simulink model "draft7"  (R2023a)
settings: Solver=VariableStepAuto  StartTime=0.0  StopTime=10  FixedStep=0.0001  MaxStep=0.1  RelTol=1e-3  AbsTol=1e-3  EnableMultiTasking=on
model workspace (MAT data in the model file):
  C_Gimbal = 0.1
  C_IAP = 0.01
  IAP_Pa = 0
  K_Gimbal = 0
  K_IAP = 10
  LeftAbdominalMuscleForce = 0
  LeftBackMuscleForce = 0
  LeftTransverse1MuscleForce = 0
  LeftTransverse2MuscleForce = 0
  Moment_AR = 0
  Moment_FE = 0
  Moment_LB = 0
  RightAbdominalMuscleForce = 0
  RightBackMuscleForce = 0
  RightTransverse1MuscleForce = 0
  RightTransverse2MuscleForce = 0
  a = 1
  b = 1
undefined symbols (not defined in the file): X, Y, Z
libraries: sm_lib x279, nesl_utility x233, simulink_extras x33, checkpacklib x3, simulink x1
(part 1 of 7)
settings Model: PacingRate=0.110000  Creator=Siril TD  LastModifiedBy=siril
settings SolverCC: AutoScaleAbsTol=off  ZeroCrossAlgorithm=Adaptive  AlgebraicLoopSolver=TrustRegion
settings DataIOCC: LimitDataPoints=on  MaxDataPoints=10000  ReturnWorkspaceOutputsName=SDOSimTest_Log
settings OptimizationCC: LifeSpan=inf
settings DebuggingCC: ReadBeforeWriteMsg=DisableAll  WriteAfterWriteMsg=DisableAll  WriteAfterReadMsg=DisableAll  IgnoredZcDiagnostic=none  MultiTaskDSMMsg=none  UnconnectedInputMsg=warning  UnconnectedOutputMsg=warning  UnconnectedLineMsg=warning  AllowSymbolicDim=off  SFUnexpectedBacktrackingDiag=warning  SFNoUnconditionalDefaultTransitionDiag=warning  SFExecutionAtInitializationDiag=none  ArithmeticOperatorsInVariantConditions=warning
settings ModelReferenceCC: EnableRefExpFcnMdlSchedulingChecks=on
settings SFSimCC: SimUseLocalCustomCode=off  CustomCodeUndefinedFunction=UseInterfaceOnly
settings RTWCC: RTWUseLocalCustomCode=off  DLArmComputeVersion=19.05
settings CodeAppCC: StateflowObjectComments=on
settings GRTTargetCC: TargetLangStandard=C89/C90 (ANSI)
settings ConfigComp: CovMetricSettings=dw  CovSaveCumulativeToWorkspaceVar=on  CovSaveSingleToWorkspaceVar=on  CovExternalEMLEnable=off  CovSFcnEnable=off
settings SimscapeCC: SimscapeLogType=all  SimscapeLogSimulationStatistics=on  SimscapeLogDataHistory=10000

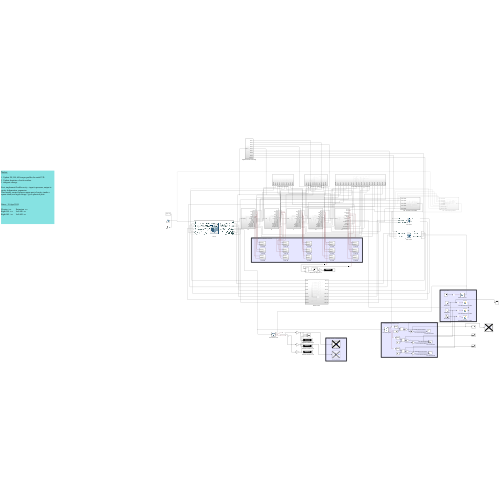
[thumbnail: Simulink's stored preview of the top-level diagram]
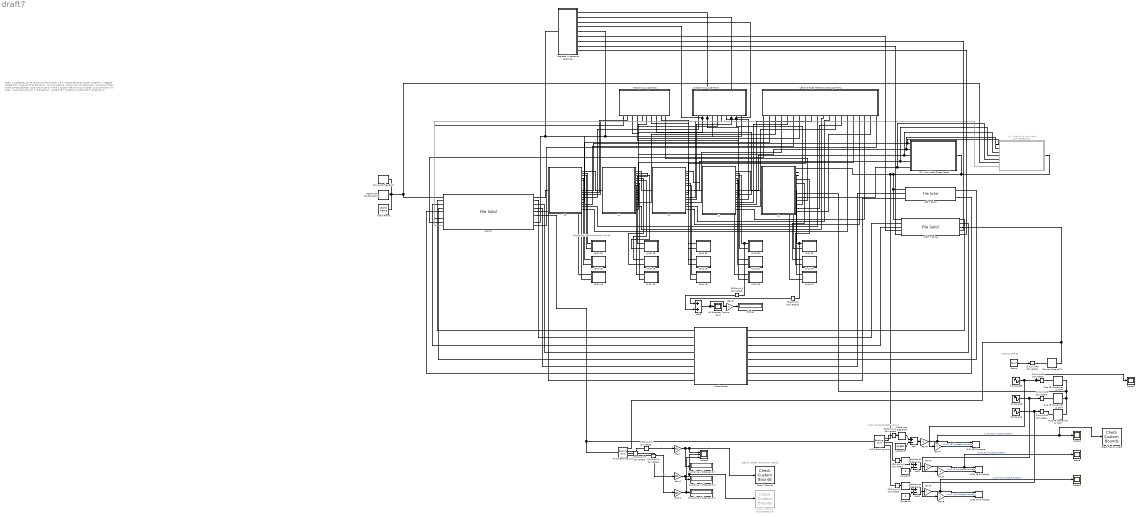
== system draft7 ==
  note: Segmental Moment-Rotation Curves
  note: L1-S1 Moment-Rotation Curve
  note: Loading Profiles
  note: Stability Check - Plumbline method
  note: Notes:
      |
      | 1. Update FE, LB, AR torque profiles for each IVD
      | 2. Update densities of each vertebra
      | 3. integrate ribcage
      |
      | First, implement flexible cavity - input is pressure, output is cavity deformation, expansion
      | Then model contact between upper part of cavity (make a square shaft) and rigid ribcage - give spherical joint
      |
      | Notes : 19-Apr-2024
      |
      | Flexion +ve Extension -ve
      | Right LB +ve Left LB -ve
      | Right AR +ve Left AR -ve
  Add : Sum  Inputs=+-
  Add1 : Sum  Inputs=+-
  Add2 : Sum  Inputs=+-
  Add3 : Sum
  Check Flexion Angle : checkpacklib/Check Custom Bounds  InstantiateOnLoad=on  enabled=off  stopWhenAssertionFail=off  export=off  ViewDlgPos=[100 200 510 390]  OpenViewOnLoad=off  LaunchViewOnOpen=off  TimeUnits=seconds  EnableUpperBound=on  UpperBoundTimes=[5 10]  UpperBoundAmplitudes=[51 51];  EnableLowerBound=on  LowerBoundTimes=[6 10]  LowerBoundAmplitudes=[49 49];
      settings: LibrarySourceBlock=sdolib/Signal Constraints/Check Custom Bounds
  Check X Bounds : checkpacklib/Check Custom Bounds  InstantiateOnLoad=on  enabled=off  stopWhenAssertionFail=off  export=off  ViewDlgPos=[622 345 510 390]  OpenViewOnLoad=off  LaunchViewOnOpen=off  TimeUnits=seconds  EnableUpperBound=on  UpperBoundTimes=[0 10]  UpperBoundAmplitudes=[2 2];  EnableLowerBound=on  LowerBoundTimes=[0 10]  LowerBoundAmplitudes=[-2 -2]
      settings: LibrarySourceBlock=sdolib/Signal Constraints/Check Custom Bounds
  Check Y Bounds : checkpacklib/Check Custom Bounds  Commented=on  InstantiateOnLoad=on  enabled=off  stopWhenAssertionFail=off  export=off  ViewDlgPos=[509 222 510 390]  OpenViewOnLoad=off  LaunchViewOnOpen=off  TimeUnits=seconds  EnableUpperBound=on  UpperBoundTimes=[0 10]  UpperBoundAmplitudes=[2 2];  EnableLowerBound=on  LowerBoundTimes=[0 10]  LowerBoundAmplitudes=[-2 -2]
      settings: LibrarySourceBlock=sdolib/Signal Constraints/Check Custom Bounds
  Constant2 : Constant  Value=14.555
  Constant3 : Constant  Value=0
  Constant4 : Constant  Value=0
  Display : Display
      settings: Decimation=2
  Flexion force at T1 : sm_lib/Forces and Torques/External Force and Torque  ForceResolutionFrame=AttachedFrame  EnableForceX=off  EnableForceY=on  EnableForceZ=off  EnableForce=off  TorqueResolutionFrame=AttachedFrame  EnableTorqueX=off  EnableTorqueY=off  EnableTorqueZ=off  EnableTorque=off
  Gain : Gain  Gain=100
  Gain1 : Gain  Gain=100
  Gain2 : Gain  Gain=100
  Gain{3..4,6..7} (4 alike) : Gain  Gain=-1
  Gain5 : Gain
  Gain8 : Gain
  Gain9 : Gain
  IAP - Individual Forces Model : Subsystem
  IAP - Internal Springs Model : Subsystem  Commented=on
  IAP Extensor Torque at L3 : Scope
  Interspinous Ligaments : Subsystem
  L1 : Subsystem
  L1-L2 AR : Subsystem
  L1-L2 FE : Subsystem
  L1-L2 LB : Subsystem
  L1-S1 AR Simscape : Record  FileSettingsInternal="{\"entries\":[{\"content\":{\"excelSettings\":{\"content\":{},\"type\":\"Streamout.ExcelSettings\"}},\"type\":\"Streamout.FileSettingStorage\",\"uuid\":\"c761fec1-51ad-4fdc-aadc-7a7c0ed1755e\"}],\"packageUris\":[\"http://schema.mathworks.com/mf0/streamout_blocks/R2020a\"],\"version\":\"1.0\"}"  Layout=[1 1]  SignalsInternal="{\"entries\":[{\"content\":{\"signals\":[{\"content\":{\"blockPath\":[\"draft7/L1-S1 AR Simscape\"],\"dimensions\":[1,1],\"domain\":\"draft7/L1-S1 AR Simscape\",\"lineColor\":\"#d95319\",\"port\":1,\"sid\":[\"\"],\"signalID\":183,\"signalName\":\"L1-S1 AR Simscape Rotation\"},\"type\":\"RecordBlkView.Signal\",\"uuid\":\"264051fc-ffd2-4aa6-9d28-74edf75983d9\"},{\"content\":{\"blockPath\":[\"draft7/L1-S1 AR Simscape\"],\"dimensions\":[1],\"domain\":\"draft7/L1-S1 AR Simscape\",\"lineColor\":\"#edb120\",\"port\":2,\"sid\":[\"\"],\"signalID\":187,\"signalName\":\"L1-S1 AR Simscape Moment\"},\"type\":\"RecordBlkView.Signal\",\"uuid\":\"a252a67f-d163-4ee1-9bea-fb1124a7b68d\"}]},\"type\":\"RecordBlkView.InputSignals\",\"uuid\":\"d04fa92a-6ab9-41c9-bd02-3e9af83bab1f\"}],\"packageUris\":[\"http://schema.mathworks.com/mf0/streamout_blocks/R2020a\"],\"version\":\"1.0\"}"  VisualizationBindings="{\"xyplotplugin\":{\"info\":[{\"series\":[],\"subplotID\":1}]}}"  CompatibilityTag=XY
  L1-S1 Bushing Joint : sm_lib/Joints/Bushing Joint  JointMode=Normal  SenseConstraintForce=off  SenseConstraintForceX=off  SenseConstraintForceY=off  SenseConstraintForceZ=off  SenseConstraintTorque=off  SenseConstraintTorqueX=off  SenseConstraintTorqueY=off  SenseConstraintTorqueZ=off  SenseTotalForce=off  SenseTotalForceX=off  SenseTotalForceY=off  SenseTotalForceZ=off  SenseTotalTorque=off  SenseTotalTorqueX=off  SenseTotalTorqueY=off  SenseTotalTorqueZ=off  CompositeWrenchDir=FollowerOnBase  CompositeWrenchFrame=FollowerFrame  PxEquilibriumPosition=0  PxEquilibriumPositionUnits=m  PxSpringStiffness=0  PxSpringStiffnessUnits=N/m  PxDampingCoefficient=0  PxDampingCoefficientUnits=N/(m/s)  PxTorqueActuationMode=NoTorque  PxMotionActuationMode=ComputedMotion  PxSensePosition=off  PxSenseVelocity=off  PxSenseAcceleration=off  PxSenseTorqueForce=off  PxSenseLowerLimitTorqueForce=off  PxSenseUpperLimitTorqueForce=off  PxLowerLimitSpecify=off  PxLowerLimitBound=-1  PxLowerLimitBoundUnits=m  PxLowerLimitStiffness=1e6  PxLowerLimitStiffnessUnits=N/m  PxLowerLimitDamping=1e3  PxLowerLimitDampingUnits=N/(m/s)  PxLowerLimitTransitionRegionWidth=1e-4  PxLowerLimitTransitionRegionWidthUnits=m  PxUpperLimitSpecify=off  PxUpperLimitBound=1  PxUpperLimitBoundUnits=m  PxUpperLimitStiffness=1e6  PxUpperLimitStiffnessUnits=N/m  PxUpperLimitDamping=1e3  PxUpperLimitDampingUnits=N/(m/s)  PxUpperLimitTransitionRegionWidth=1e-4  PxUpperLimitTransitionRegionWidthUnits=m  PxPositionTargetSpecify=off  PxPositionTargetPriority=High  PxPositionTargetValue=0  PxPositionTargetValueUnits=m  PxVelocityTargetSpecify=off  PxVelocityTargetPriority=High  PxVelocityTargetValue=0  PxVelocityTargetValueUnits=m/s  PyEquilibriumPosition=0  PyEquilibriumPositionUnits=m  PySpringStiffness=0  PySpringStiffnessUnits=N/m  PyDampingCoefficient=0  PyDampingCoefficientUnits=N/(m/s)  PyTorqueActuationMode=NoTorque  PyMotionActuationMode=ComputedMotion  PySensePosition=off  PySenseVelocity=off  PySenseAcceleration=off  PySenseTorqueForce=off  PySenseLowerLimitTorqueForce=off  PySenseUpperLimitTorqueForce=off  PyLowerLimitSpecify=off  PyLowerLimitBound=-1  PyLowerLimitBoundUnits=m  PyLowerLimitStiffness=1e6  PyLowerLimitStiffnessUnits=N/m  PyLowerLimitDamping=1e3  PyLowerLimitDampingUnits=N/(m/s)  PyLowerLimitTransitionRegionWidth=1e-4  PyLowerLimitTransitionRegionWidthUnits=m  PyUpperLimitSpecify=off  PyUpperLimitBound=1  PyUpperLimitBoundUnits=m  PyUpperLimitStiffness=1e6  PyUpperLimitStiffnessUnits=N/m  PyUpperLimitDamping=1e3  PyUpperLimitDampingUnits=N/(m/s)  PyUpperLimitTransitionRegionWidth=1e-4  PyUpperLimitTransitionRegionWidthUnits=m  PyPositionTargetSpecify=off  PyPositionTargetPriority=High  PyPositionTargetValue=0  PyPositionTargetValueUnits=m  PyVelocityTargetSpecify=off  PyVelocityTargetPriority=High  PyVelocityTargetValue=0  PyVelocityTargetValueUnits=m/s  PzEquilibriumPosition=0  PzEquilibriumPositionUnits=m  PzSpringStiffness=0  PzSpringStiffnessUnits=N/m  PzDampingCoefficient=0  PzDampingCoefficientUnits=N/(m/s)  PzTorqueActuationMode=NoTorque  PzMotionActuationMode=ComputedMotion  PzSensePosition=off  PzSenseVelocity=off  PzSenseAcceleration=off  PzSenseTorqueForce=off  PzSenseLowerLimitTorqueForce=off  PzSenseUpperLimitTorqueForce=off  PzLowerLimitSpecify=off  PzLowerLimitBound=-1  PzLowerLimitBoundUnits=m  PzLowerLimitStiffness=1e6  PzLowerLimitStiffnessUnits=N/m  PzLowerLimitDamping=1e3  PzLowerLimitDampingUnits=N/(m/s)  PzLowerLimitTransitionRegionWidth=1e-4  PzLowerLimitTransitionRegionWidthUnits=m  PzUpperLimitSpecify=off  PzUpperLimitBound=1  PzUpperLimitBoundUnits=m  PzUpperLimitStiffness=1e6  PzUpperLimitStiffnessUnits=N/m  PzUpperLimitDamping=1e3  PzUpperLimitDampingUnits=N/(m/s)  PzUpperLimitTransitionRegionWidth=1e-4  PzUpperLimitTransitionRegionWidthUnits=m  PzPositionTargetSpecify=off  PzPositionTargetPriority=High  PzPositionTargetValue=0  PzPositionTargetValueUnits=m  PzVelocityTargetSpecify=off  PzVelocityTargetPriority=High  PzVelocityTargetValue=0  PzVelocityTargetValueUnits=m/s  RxEquilibriumPosition=0  RxEquilibriumPositionUnits=deg  RxSpringStiffness=0  RxSpringStiffnessUnits=N*m/deg  RxDampingCoefficient=0  RxDampingCoefficientUnits=N*m/(deg/s)  RxTorqueActuationMode=NoTorque  RxMotionActuationMode=ComputedMotion  RxSensePosition=on  RxSenseVelocity=off  RxSenseAcceleration=off  RxSenseTorqueForce=off  RxSenseLowerLimitTorqueForce=off  RxSenseUpperLimitTorqueForce=off  RxLowerLimitSpecify=off  RxLowerLimitBound=-90  RxLowerLimitBoundUnits=deg  RxLowerLimitStiffness=1e4  RxLowerLimitStiffnessUnits=N*m/deg  RxLowerLimitDamping=10  RxLowerLimitDampingUnits=N*m/(deg/s)  RxLowerLimitTransitionRegionWidth=0.1  RxLowerLimitTransitionRegionWidthUnits=deg  RxUpperLimitSpecify=off  RxUpperLimitBound=90  RxUpperLimitBoundUnits=deg  RxUpperLimitStiffness=1e4  RxUpperLimitStiffnessUnits=N*m/deg  RxUpperLimitDamping=10  RxUpperLimitDampingUnits=N*m/(deg/s)  RxUpperLimitTransitionRegionWidth=0.1  RxUpperLimitTransitionRegionWidthUnits=deg  RxPositionTargetSpecify=off  RxPositionTargetPriority=High  RxPositionTargetValue=0  RxPositionTargetValueUnits=deg  RxVelocityTargetSpecify=off  RxVelocityTargetPriority=High  RxVelocityTargetValue=0  RxVelocityTargetValueUnits=deg/s  RyEquilibriumPosition=0  RyEquilibriumPositionUnits=deg  RySpringStiffness=0  RySpringStiffnessUnits=N*m/deg  RyDampingCoefficient=0  RyDampingCoefficientUnits=N*m/(deg/s)  RyTorqueActuationMode=NoTorque  RyMotionActuationMode=ComputedMotion  RySensePosition=on  RySenseVelocity=off  RySenseAcceleration=off  RySenseTorqueForce=off  RySenseLowerLimitTorqueForce=off  RySenseUpperLimitTorqueForce=off  RyLowerLimitSpecify=off  RyLowerLimitBound=-90  RyLowerLimitBoundUnits=deg  RyLowerLimitStiffness=1e4  RyLowerLimitStiffnessUnits=N*m/deg  RyLowerLimitDamping=10  RyLowerLimitDampingUnits=N*m/(deg/s)  RyLowerLimitTransitionRegionWidth=0.1  RyLowerLimitTransitionRegionWidthUnits=deg  RyUpperLimitSpecify=off  RyUpperLimitBound=90  RyUpperLimitBoundUnits=deg  RyUpperLimitStiffness=1e4  RyUpperLimitStiffnessUnits=N*m/deg  RyUpperLimitDamping=10  RyUpperLimitDampingUnits=N*m/(deg/s)  RyUpperLimitTransitionRegionWidth=0.1  RyUpperLimitTransitionRegionWidthUnits=deg  RyPositionTargetSpecify=off  RyPositionTargetPriority=High  RyPositionTargetValue=0  RyPositionTargetValueUnits=deg  RyVelocityTargetSpecify=off  RyVelocityTargetPriority=High  RyVelocityTargetValue=0  RyVelocityTargetValueUnits=deg/s  RzEquilibriumPosition=0  RzEquilibriumPositionUnits=deg  RzSpringStiffness=0  RzSpringStiffnessUnits=N*m/deg  RzDampingCoefficient=0  RzDampingCoefficientUnits=N*m/(deg/s)  RzTorqueActuationMode=NoTorque  RzMotionActuationMode=ComputedMotion  RzSensePosition=on  RzSenseVelocity=off  RzSenseAcceleration=off  RzSenseTorqueForce=off  RzSenseLowerLimitTorqueForce=off  RzSenseUpperLimitTorqueForce=off  RzLowerLimitSpecify=off  RzLowerLimitBound=-90  RzLowerLimitBoundUnits=deg  RzLowerLimitStiffness=1e4  RzLowerLimitStiffnessUnits=N*m/deg  RzLowerLimitDamping=10  RzLowerLimitDampingUnits=N*m/(deg/s)  RzLowerLimitTransitionRegionWidth=0.1  RzLowerLimitTransitionRegionWidthUnits=deg  RzUpperLimitSpecify=off  RzUpperLimitBound=90  RzUpperLimitBoundUnits=deg  RzUpperLimitStiffness=1e4  RzUpperLimitStiffnessUnits=N*m/deg  RzUpperLimitDamping=10  RzUpperLimitDampingUnits=N*m/(deg/s)  RzUpperLimitTransitionRegionWidth=0.1  RzUpperLimitTransitionRegionWidthUnits=deg  RzPositionTargetSpecify=off  RzPositionTargetPriority=High  RzPositionTargetValue=0  RzPositionTargetValueUnits=deg  RzVelocityTargetSpecify=off  RzVelocityTargetPriority=High  RzVelocityTargetValue=0  RzVelocityTargetValueUnits=deg/s
  L1-S1 FE Simscape : Record  FileSettingsInternal="{\"entries\":[{\"content\":{\"excelSettings\":{\"content\":{},\"type\":\"Streamout.ExcelSettings\"}},\"type\":\"Streamout.FileSettingStorage\",\"uuid\":\"9db1673e-bbaa-437a-8537-4e772d2a90f6\"}],\"packageUris\":[\"http://schema.mathworks.com/mf0/streamout_blocks/R2020a\"],\"version\":\"1.0\"}"  Layout=[1 1]  SignalsInternal="{\"entries\":[{\"content\":{\"signals\":[{\"content\":{\"blockPath\":[\"draft7/L1-S1 FE Simscape\"],\"dimensions\":[1,1],\"domain\":\"draft7/L1-S1 FE Simscape\",\"lineColor\":\"#ff13a6\",\"port\":1,\"sid\":[\"\"],\"signalID\":167,\"signalName\":\"L1-S1 FE Simscape Rotation\"},\"type\":\"RecordBlkView.Signal\",\"uuid\":\"c1594988-5f2b-4ea3-9ef2-5b94fe21d5f8\"},{\"content\":{\"blockPath\":[\"draft7/L1-S1 FE Simscape\"],\"dimensions\":[1],\"domain\":\"draft7/L1-S1 FE Simscape\",\"lineColor\":\"#fe330a\",\"port\":2,\"sid\":[\"\"],\"signalID\":171,\"signalName\":\"L1-S1 FE Simscape Moment\"},\"type\":\"RecordBlkView.Signal\",\"uuid\":\"b92ce8fd-0f35-4184-b4f5-937e9b6e7470\"}]},\"type\":\"RecordBlkView.InputSignals\",\"uuid\":\"db540f72-e83b-464a-95e3-44d444f527ba\"}],\"packageUris\":[\"http://schema.mathworks.com/mf0/streamout_blocks/R2020a\"],\"version\":\"1.0\"}"  VisualizationBindings="{\"xyplotplugin\":{\"info\":[{\"series\":[],\"subplotID\":1}]}}"  CompatibilityTag=XY
  L1-S1 LB Simscape : Record  FileSettingsInternal="{\"entries\":[{\"content\":{\"excelSettings\":{\"content\":{},\"type\":\"Streamout.ExcelSettings\"}},\"type\":\"Streamout.FileSettingStorage\",\"uuid\":\"68995d24-6116-4abf-89ba-75caefee83bb\"}],\"packageUris\":[\"http://schema.mathworks.com/mf0/streamout_blocks/R2020a\"],\"version\":\"1.0\"}"  Layout=[1 1]  SignalsInternal="{\"entries\":[{\"content\":{\"signals\":[{\"content\":{\"blockPath\":[\"draft7/L1-S1 LB Simscape\"],\"dimensions\":[1,1],\"domain\":\"draft7/L1-S1 LB Simscape\",\"lineColor\":\"#22b573\",\"port\":1,\"sid\":[\"\"],\"signalID\":175,\"signalName\":\"L1-S1 LB Simscape Rotation\"},\"type\":\"RecordBlkView.Signal\",\"uuid\":\"30783bb8-1c86-4cdf-87e2-2a28f747091a\"},{\"content\":{\"blockPath\":[\"draft7/L1-S1 LB Simscape\"],\"dimensions\":[1],\"domain\":\"draft7/L1-S1 LB Simscape\",\"lineColor\":\"#0072bd\",\"port\":2,\"sid\":[\"\"],\"signalID\":179,\"signalName\":\"L1-S1 LB Simscape Moment\"},\"type\":\"RecordBlkView.Signal\",\"uuid\":\"2a8f21ee-91f9-4dc2-9379-b6999c3c9a9c\"}]},\"type\":\"RecordBlkView.InputSignals\",\"uuid\":\"a080d18d-00c5-434d-a6df-27a9e497c067\"}],\"packageUris\":[\"http://schema.mathworks.com/mf0/streamout_blocks/R2020a\"],\"version\":\"1.0\"}"  VisualizationBindings="{\"xyplotplugin\":{\"info\":[{\"series\":[],\"subplotID\":1}]}}"  CompatibilityTag=XY
  L2 : Subsystem
  L2-L3 AR : Subsystem
  L2-L3 FE : Subsystem
  L2-L3 LB : Subsystem
  L3 : Subsystem
  L3-L4 AR : Subsystem
  L3-L4 FE : Subsystem
  L3-L4 LB : Subsystem
  L4 : Subsystem
  L4-L5  AR : Subsystem
  L4-L5  FE : Subsystem
  L4-L5  LB : Subsystem
  L5 : Subsystem
  L5-S1 AR : Subsystem
  L5-S1 FE : Subsystem
  L5-S1 LB : Subsystem
  Left T Spine : sm_lib/Body Elements/File Solid  ExtGeomFileName=C:\Users\siril\OneDrive\Desktop\TIM-Control\Matlab\Simscape models\CAD - with COM\SymmetricModel\draft7\LeftThoracicSpineWithRibcage.step  UnitType=FromFile  ExtGeomFileUnits=m  StepReaderType=HEX  ExportConvexHullGeometry=off  InertiaType=CalculateFromGeometry  Mass=1  MassUnits=kg  CenterOfMass=[0 0 0]  CenterOfMassUnits=m  MomentsOfInertia=[1 1 1]  MomentsOfInertiaUnits=kg*m^2  ProductsOfInertia=[0 0 0]  ProductsOfInertiaUnits=kg*m^2  BasedOnType=Density  Density=0.182  DensityUnits=g/cm^3  DoExposeReferenceFrame=off  SerializedFrames=<Frames><Frame><Id>Frame1</Id><Value><Name>To L1</Name><Origin><Source>GeometricFeature</Source><FeatureName>segment 762</FeatureName></Origin><PrimaryAxis><DefinedDirection>-Z</DefinedDirection><Source>GeometricFeature</Source><SourceDirection>+Z</SourceDirection><FeatureName>planar surface 1266</FeatureName></PrimaryAxis><SecondaryAxis><DefinedDirection>+X</DefinedDirection><Source>ReferenceFrame</Source><SourceDirection>+X</SourceDirection><FeatureName></FeatureName></SecondaryAxis></Value></Frame><Frame><Id>Frame2</Id><Value><Name>To Left Abdominal Muscle</Name><Origin><Source>GeometricFeature</Source><FeatureName>planar surface 54556</FeatureName></Origin><PrimaryAxis><DefinedDirection>+Z</DefinedDirection><Source>GeometricFeature</Source><SourceDirection>+Z</SourceDirection><FeatureName>planar surface 54556</FeatureName></PrimaryAxis><SecondaryAxis><DefinedDirection>+X</DefinedDirection><Source>ReferenceFrame</Source><SourceDirection>+X</SourceDirection><FeatureName></FeatureName></SecondaryAxis></Value></Frame><Frame><Id>Frame3</Id><Value><Name>To Left Back Muscle</Name><Origin><Source>GeometricFeature</Source><FeatureName>planar surface 54574</FeatureName></Origin><PrimaryAxis><DefinedDirection>-Z</DefinedDirection><Source>GeometricFeature</Source><SourceDirection>+Z</SourceDirection><FeatureName>planar surface 54574</FeatureName></PrimaryAxis><SecondaryAxis><DefinedDirection>+X</DefinedDirection><Source>ReferenceFrame</Source><SourceDirection>+X</SourceDirection><FeatureName></FeatureName></SecondaryAxis></Value></Frame><Frame><Id>Frame4</Id><Value><Name>To Left Transverse1 Muscle</Name><Origin><Source>GeometricFeature</Source><FeatureName>planar surface 54586</FeatureName></Origin><PrimaryAxis><DefinedDirection>+Z</DefinedDirection><Source>GeometricFeature</Source><SourceDirection>+Z</SourceDirection><FeatureName>planar surface 54586</FeatureName></PrimaryAxis><SecondaryAxis><DefinedDirection>+X</DefinedDirection><Source>ReferenceFrame</Source><SourceDirection>+X</SourceDirection><FeatureName></FeatureName></SecondaryAxis></Value></Frame><Frame><Id>Frame5</Id><Value><Name>To Left Transverse2 Muscle</Name><Origin><Source>GeometricFeature</Source><FeatureName>planar surface 54611</FeatureName></Origin><PrimaryAxis><DefinedDirection>+Z</DefinedDirection><Source>GeometricFeature</Source><SourceDirection>+Z</SourceDirection><FeatureName>planar surface 54611</FeatureName></PrimaryAxis><SecondaryAxis><DefinedDirection>+X</DefinedDirection><Source>ReferenceFrame</Source><SourceDirection>+X</SourceDirection><FeatureName></FeatureName></SecondaryAxis></Value></Frame></Frames>  GraphicType=FromGeometry  MarkerShape=Sphere  MarkerSize=10  GraphicVisPropType=SimpleVisualProperties  GraphicDiffuseColor=[0.5 0.5 0.5]  GraphicSpecularColor=[0.5 0.5 0.5 1.0]  GraphicAmbientColor=[0.15 0.15 0.15 1.0]  GraphicEmissiveColor=[0.0 0.0 0.0 1.0]  GraphicShininess=75  GraphicOpacity=1.0
  Left and Right Intertransverse Ligaments : Subsystem
  Mechanism Configuration : sm_lib/Utilities/Mechanism Configuration  UniformGravity=Constant  GravityVector=[0 0 -9.80665]  GravityVectorUnits=m/s^2  LinearizationDelta=0.001  JointModeTransitionNonlinearIterations=2
  Moment_AR : Sin  Amplitude=Moment_AR  SampleTime=0
  Moment_FE : Sin  Amplitude=-Moment_FE  SampleTime=0
  Moment_LB : Sin  Amplitude=-Moment_LB  SampleTime=0
  Muscle Forces : Subsystem
  PS-Simulink Converter{1..5,8..10} (8 alike) : nesl_utility/PS-Simulink Converter  PhysicalDomain=network_engine_domain  SubClassName=ps_output  LeftPortType=input  RightPortType=output  PseudoPeriodic=off  Frequencies=[]  VectorFormat=inherit  Unit=inherit  AffineConversion=off
  Plumbline X distance (cm) : Display
  Plumbline Y distance (cm) : Display
  Plumbline Z distance (cm) : Display
  Pure AR Moment at L1 COM : sm_lib/Forces and Torques/External Force and Torque  ForceResolutionFrame=World  EnableForceX=off  EnableForceY=off  EnableForceZ=off  EnableForce=off  TorqueResolutionFrame=World  EnableTorqueX=off  EnableTorqueY=off  EnableTorqueZ=on  EnableTorque=off
  Pure FE Moment at L1 COM : sm_lib/Forces and Torques/External Force and Torque  ForceResolutionFrame=World  EnableForceX=off  EnableForceY=off  EnableForceZ=off  EnableForce=off  TorqueResolutionFrame=World  EnableTorqueX=on  EnableTorqueY=off  EnableTorqueZ=off  EnableTorque=off
  Pure LB Moment at L1 COM : sm_lib/Forces and Torques/External Force and Torque  ForceResolutionFrame=World  EnableForceX=off  EnableForceY=off  EnableForceZ=off  EnableForce=off  TorqueResolutionFrame=World  EnableTorqueX=off  EnableTorqueY=on  EnableTorqueZ=off  EnableTorque=off
  Radians to Degrees1 : simulink_extras/Transformations/Radians to Degrees
  Radians to Degrees2 : simulink_extras/Transformations/Radians to Degrees
  Radians to Degrees4 : simulink_extras/Transformations/Radians to Degrees
  Ramp : simulink/Sources/Ramp  slope=0  start=0  InitialOutput=0
  Right T Spine : sm_lib/Body Elements/File Solid  ExtGeomFileName=C:\Users\siril\OneDrive\Desktop\TIM-Control\Matlab\Simscape models\CAD - with COM\SymmetricModel\draft7\RightThoracicSpineWithRibcage.step  UnitType=FromFile  ExtGeomFileUnits=m  StepReaderType=HEX  ExportConvexHullGeometry=off  InertiaType=CalculateFromGeometry  Mass=1  MassUnits=kg  CenterOfMass=[0 0 0]  CenterOfMassUnits=m  MomentsOfInertia=[1 1 1]  MomentsOfInertiaUnits=kg*m^2  ProductsOfInertia=[0 0 0]  ProductsOfInertiaUnits=kg*m^2  BasedOnType=Density  Density=0.182  DensityUnits=g/cm^3  DoExposeReferenceFrame=off  SerializedFrames=<Frames><Frame><Id>Frame1</Id><Value><Name>To L1</Name><Origin><Source>GeometricFeature</Source><FeatureName>segment 633</FeatureName></Origin><PrimaryAxis><DefinedDirection>+Z</DefinedDirection><Source>GeometricFeature</Source><SourceDirection>+Z</SourceDirection><FeatureName>planar surface 1266</FeatureName></PrimaryAxis><SecondaryAxis><DefinedDirection>+X</DefinedDirection><Source>ReferenceFrame</Source><SourceDirection>+X</SourceDirection><FeatureName></FeatureName></SecondaryAxis></Value></Frame><Frame><Id>Frame2</Id><Value><Name>To Right Abdominal Muscle</Name><Origin><Source>GeometricFeature</Source><FeatureName>planar surface 54556</FeatureName></Origin><PrimaryAxis><DefinedDirection>-Z</DefinedDirection><Source>GeometricFeature</Source><SourceDirection>+Z</SourceDirection><FeatureName>planar surface 54556</FeatureName></PrimaryAxis><SecondaryAxis><DefinedDirection>+X</DefinedDirection><Source>ReferenceFrame</Source><SourceDirection>+X</SourceDirection><FeatureName></FeatureName></SecondaryAxis></Value></Frame><Frame><Id>Frame3</Id><Value><Name>To Right Back Muscle</Name><Origin><Source>GeometricFeature</Source><FeatureName>planar surface 54574</FeatureName></Origin><PrimaryAxis><DefinedDirection>+Z</DefinedDirection><Source>GeometricFeature</Source><SourceDirection>+Z</SourceDirection><FeatureName>planar surface 54574</FeatureName></PrimaryAxis><SecondaryAxis><DefinedDirection>+X</DefinedDirection><Source>ReferenceFrame</Source><SourceDirection>+X</SourceDirection><FeatureName></FeatureName></SecondaryAxis></Value></Frame><Frame><Id>Frame4</Id><Value><Name>To Right Transverse1 Muscle</Name><Origin><Source>GeometricFeature</Source><FeatureName>planar surface 54586</FeatureName></Origin><PrimaryAxis><DefinedDirection>-Z</DefinedDirection><Source>GeometricFeature</Source><SourceDirection>+Z</SourceDirection><FeatureName>planar surface 54586</FeatureName></PrimaryAxis><SecondaryAxis><DefinedDirection>+X</DefinedDirection><Source>ReferenceFrame</Source><SourceDirection>+X</SourceDirection><FeatureName></FeatureName></SecondaryAxis></Value></Frame><Frame><Id>Frame5</Id><Value><Name>To Right Transverse2 Muscle</Name><Origin><Source>GeometricFeature</Source><FeatureName>planar surface 54611</FeatureName></Origin><PrimaryAxis><DefinedDirection>-Z</DefinedDirection><Source>GeometricFeature</Source><SourceDirection>+Z</SourceDirection><FeatureName>planar surface 54611</FeatureName></PrimaryAxis><SecondaryAxis><DefinedDirection>+X</DefinedDirection><Source>ReferenceFrame</Source><SourceDirection>+X</SourceDirection><FeatureName></FeatureName></SecondaryAxis></Value></Frame><Frame><Id>Frame6</Id><Value><Name>T1 Plumbline Frame</Name><Origin><Source>GeometricFeature</Source><FeatureName>point 5793</FeatureName></Origin><PrimaryAxis><DefinedDirection>+Z</DefinedDirection><Source>ReferenceFrame</Source><SourceDirection>+Z</SourceDirection><FeatureName></FeatureName></PrimaryAxis><SecondaryAxis><DefinedDirection>+X</DefinedDirection><Source>ReferenceFrame</Source><SourceDirection>+X</SourceDirection><FeatureName></FeatureName></SecondaryAxis></Value></Frame><Frame><Id>Frame7</Id><Value><Name>T5 Spinous Process Tip</Name><Origin><Source>GeometricFeature</Source><FeatureName>point 6426</FeatureName></Origin><PrimaryAxis><DefinedDirection>+Z</DefinedDirection><Source>ReferenceFrame</Source><SourceDirection>+Z</SourceDirection><FeatureName></FeatureName></PrimaryAxis><SecondaryAxis><DefinedDirection>+X</DefinedDirection><Source>ReferenceFrame</Source><SourceDirection>+X</SourceDirection><FeatureName></FeatureName></SecondaryAxis></Value></Frame><Frame><Id>Frame8</Id><Value><Name>T1 Spinous Process Tip</Name><Origin><Source>GeometricFeature</Source><FeatureName>point 327</FeatureName></Origin><PrimaryAxis><DefinedDirection>+Z</DefinedDirection><Source>ReferenceFrame</Source><SourceDirection>+Z</SourceDirection><FeatureName></FeatureName></PrimaryAxis><SecondaryAxis><DefinedDirection>+X</DefinedDirection><Source>ReferenceFrame</Source><SourceDirection>+X</SourceDirection><FeatureName></FeatureName></SecondaryAxis></Value></Frame><Frame><Id>Frame9</Id><Value><Name>T10 Spinous process tip</Name><Origin><Source>GeometricFeature</Source><FeatureName>point 46212</FeatureName></Origin><PrimaryAxis><DefinedDirection>+Z</DefinedDirection><Source>ReferenceFrame</Source><SourceDirection>+Z</SourceDirection><FeatureName></FeatureName></PrimaryAxis><SecondaryAxis><DefinedDirection>+X</DefinedDirection><Source>ReferenceFrame</Source><SourceDirection>+X</SourceDirection><FeatureName></FeatureName></SecondaryAxis></Value></Frame><Frame><Id>Frame10</Id><Value><Name>T12 Spinous Process tip</Name><Origin><Source>GeometricFeature</Source><FeatureName>point 4338</FeatureName></Origin><PrimaryAxis><DefinedDirection>+Z</DefinedDirection><Source>ReferenceFrame</Source><SourceDirection>+Z</SourceDirection><FeatureName></FeatureName></PrimaryAxis><SecondaryAxis><DefinedDirection>+X</DefinedDirection><Source>ReferenceFrame</Source><SourceDirection>+X</SourceDirection><FeatureName></FeatureName></SecondaryAxis></Value></Frame></Frames>  GraphicType=FromGeometry  MarkerShape=Sphere  MarkerSize=10  GraphicVisPropType=SimpleVisualProperties  GraphicDiffuseColor=[0.5 0.5 0.5]  GraphicSpecularColor=[0.5 0.5 0.5 1.0]  GraphicAmbientColor=[0.15 0.15 0.15 1.0]  GraphicEmissiveColor=[0.0 0.0 0.0 1.0]  GraphicShininess=75  GraphicOpacity=1.0
  Sagittaal Kinematics Readings : Subsystem
  Scope{,1..3} (4 alike) : Scope
  Scope9 : Scope  NumInputPorts=3
  Simulink-PS Converter{1..4} (4 alike) : nesl_utility/Simulink-PS Converter  PhysicalDomain=network_engine_domain  SubClassName=ps_input  LeftPortType=input  RightPortType=output  PseudoPeriodic=off  Frequencies=[]  NoiseDistribution=none  NoiseParameters=[]  Unit=1  AffineConversion=off  FilteringAndDerivatives=provide  SimscapeFilterOrder=1  InputFilterTimeConstant=0.001  UdotUserProvided=0
  Solver Configuration : nesl_utility/Solver Configuration  PhysicalDomain=network_engine_domain  SubClassName=solver  LeftPortType=input  RightPortType=generic  Tones=[]  Harmonics=[]  SimulateNoise=off  Profile=off  UseLocalSampling=off  EnableSwitchedLinearOptims=on  FrequencyDomain=off  UseCCode=off  RelTol=0.001  AbsTol=1e-06  MinStep=1e-09  ToWorkspace=off  RevertToSquareIcSolve=off  NumHomotopyIterations=100  PhasorMode=off  PhasorModeNumHarmonics=1  ConsistencySolver=NEWTON_FTOL  IndexReductionMethod=DerivativeReplacement  DoDC=off  ResidualTolerance=1e-09  ConsistencyTolSource=GLOBAL  ConsistencyAbsTol=0.001  ConsistencyRelTol=0.001  ConsistencyTolFactor=0.001  UseLocalSolver=off  LocalSolverChoice=NE_BACKWARD_EULER_ADVANCER  ResolveIndetEquations=on  FunctionEvalNumThread=1  LocalSolverSampleTime=0.001  DoFixedCost=off  MaxNonlinIter=3  MaxModeIter=2  ComputeImpulses=off  ImpulseIterations=2  LinearAlgebra=Sparse  LinearAlgebraNumThread=0  EquationFormulation=NE_TIME_EF  DelaysMemoryBudget=1024  AutomaticFiltering=on  FilteringTimeConstant=0.001  PartitionStorageMethod=AS_NEEDED  PartitionMemoryBudget=1024  PartitionMethod=FAST
  Supraspinous Ligaments : Subsystem
  T1-S1 Bushing Joint : sm_lib/Joints/Bushing Joint  JointMode=Normal  SenseConstraintForce=off  SenseConstraintForceX=off  SenseConstraintForceY=off  SenseConstraintForceZ=off  SenseConstraintTorque=off  SenseConstraintTorqueX=off  SenseConstraintTorqueY=off  SenseConstraintTorqueZ=off  SenseTotalForce=off  SenseTotalForceX=off  SenseTotalForceY=off  SenseTotalForceZ=off  SenseTotalTorque=off  SenseTotalTorqueX=off  SenseTotalTorqueY=off  SenseTotalTorqueZ=off  CompositeWrenchDir=FollowerOnBase  CompositeWrenchFrame=BaseFrame  PxEquilibriumPosition=0  PxEquilibriumPositionUnits=m  PxSpringStiffness=0  PxSpringStiffnessUnits=N/m  PxDampingCoefficient=0  PxDampingCoefficientUnits=N/(m/s)  PxTorqueActuationMode=NoTorque  PxMotionActuationMode=ComputedMotion  PxSensePosition=on  PxSenseVelocity=off  PxSenseAcceleration=off  PxSenseTorqueForce=off  PxSenseLowerLimitTorqueForce=off  PxSenseUpperLimitTorqueForce=off  PxLowerLimitSpecify=off  PxLowerLimitBound=-1  PxLowerLimitBoundUnits=m  PxLowerLimitStiffness=1e6  PxLowerLimitStiffnessUnits=N/m  PxLowerLimitDamping=1e3  PxLowerLimitDampingUnits=N/(m/s)  PxLowerLimitTransitionRegionWidth=1e-4  PxLowerLimitTransitionRegionWidthUnits=m  PxUpperLimitSpecify=off  PxUpperLimitBound=1  PxUpperLimitBoundUnits=m  PxUpperLimitStiffness=1e6  PxUpperLimitStiffnessUnits=N/m  PxUpperLimitDamping=1e3  PxUpperLimitDampingUnits=N/(m/s)  PxUpperLimitTransitionRegionWidth=1e-4  PxUpperLimitTransitionRegionWidthUnits=m  PxPositionTargetSpecify=off  PxPositionTargetPriority=High  PxPositionTargetValue=0  PxPositionTargetValueUnits=m  PxVelocityTargetSpecify=off  PxVelocityTargetPriority=High  PxVelocityTargetValue=0  PxVelocityTargetValueUnits=m/s  PyEquilibriumPosition=0  PyEquilibriumPositionUnits=m  PySpringStiffness=0  PySpringStiffnessUnits=N/m  PyDampingCoefficient=0  PyDampingCoefficientUnits=N/(m/s)  PyTorqueActuationMode=NoTorque  PyMotionActuationMode=ComputedMotion  PySensePosition=on  PySenseVelocity=off  PySenseAcceleration=off  PySenseTorqueForce=off  PySenseLowerLimitTorqueForce=off  PySenseUpperLimitTorqueForce=off  PyLowerLimitSpecify=off  PyLowerLimitBound=-1  PyLowerLimitBoundUnits=m  PyLowerLimitStiffness=1e6  PyLowerLimitStiffnessUnits=N/m  PyLowerLimitDamping=1e3  PyLowerLimitDampingUnits=N/(m/s)  PyLowerLimitTransitionRegionWidth=1e-4  PyLowerLimitTransitionRegionWidthUnits=m  PyUpperLimitSpecify=off  PyUpperLimitBound=1  PyUpperLimitBoundUnits=m  PyUpperLimitStiffness=1e6  PyUpperLimitStiffnessUnits=N/m  PyUpperLimitDamping=1e3  PyUpperLimitDampingUnits=N/(m/s)  PyUpperLimitTransitionRegionWidth=1e-4  PyUpperLimitTransitionRegionWidthUnits=m  PyPositionTargetSpecify=off  PyPositionTargetPriority=High  PyPositionTargetValue=0  PyPositionTargetValueUnits=m  PyVelocityTargetSpecify=off  PyVelocityTargetPriority=High  PyVelocityTargetValue=0  PyVelocityTargetValueUnits=m/s  PzEquilibriumPosition=0  PzEquilibriumPositionUnits=m  PzSpringStiffness=0  PzSpringStiffnessUnits=N/m  PzDampingCoefficient=0  PzDampingCoefficientUnits=N/(m/s)  PzTorqueActuationMode=NoTorque  PzMotionActuationMode=ComputedMotion  PzSensePosition=on  PzSenseVelocity=off  PzSenseAcceleration=off  PzSenseTorqueForce=off  PzSenseLowerLimitTorqueForce=off  PzSenseUpperLimitTorqueForce=off  PzLowerLimitSpecify=off  PzLowerLimitBound=-1  PzLowerLimitBoundUnits=m  PzLowerLimitStiffness=1e6  PzLowerLimitStiffnessUnits=N/m  PzLowerLimitDamping=1e3  PzLowerLimitDampingUnits=N/(m/s)  PzLowerLimitTransitionRegionWidth=1e-4  PzLowerLimitTransitionRegionWidthUnits=m  PzUpperLimitSpecify=off  PzUpperLimitBound=1  PzUpperLimitBoundUnits=m  PzUpperLimitStiffness=1e6  PzUpperLimitStiffnessUnits=N/m  PzUpperLimitDamping=1e3  PzUpperLimitDampingUnits=N/(m/s)  PzUpperLimitTransitionRegionWidth=1e-4  PzUpperLimitTransitionRegionWidthUnits=m  PzPositionTargetSpecify=off  PzPositionTargetPriority=High  PzPositionTargetValue=0  PzPositionTargetValueUnits=m  PzVelocityTargetSpecify=off  PzVelocityTargetPriority=High  PzVelocityTargetValue=0  PzVelocityTargetValueUnits=m/s  RxEquilibriumPosition=0  RxEquilibriumPositionUnits=deg  RxSpringStiffness=0  RxSpringStiffnessUnits=N*m/deg  RxDampingCoefficient=0  RxDampingCoefficientUnits=N*m/(deg/s)  RxTorqueActuationMode=NoTorque  RxMotionActuationMode=ComputedMotion  RxSensePosition=off  RxSenseVelocity=off  RxSenseAcceleration=off  RxSenseTorqueForce=off  RxSenseLowerLimitTorqueForce=off  RxSenseUpperLimitTorqueForce=off  RxLowerLimitSpecify=off  RxLowerLimitBound=-90  RxLowerLimitBoundUnits=deg  RxLowerLimitStiffness=1e4  RxLowerLimitStiffnessUnits=N*m/deg  RxLowerLimitDamping=10  RxLowerLimitDampingUnits=N*m/(deg/s)  RxLowerLimitTransitionRegionWidth=0.1  RxLowerLimitTransitionRegionWidthUnits=deg  RxUpperLimitSpecify=off  RxUpperLimitBound=90  RxUpperLimitBoundUnits=deg  RxUpperLimitStiffness=1e4  RxUpperLimitStiffnessUnits=N*m/deg  RxUpperLimitDamping=10  RxUpperLimitDampingUnits=N*m/(deg/s)  RxUpperLimitTransitionRegionWidth=0.1  RxUpperLimitTransitionRegionWidthUnits=deg  RxPositionTargetSpecify=off  RxPositionTargetPriority=High  RxPositionTargetValue=0  RxPositionTargetValueUnits=deg  RxVelocityTargetSpecify=off  RxVelocityTargetPriority=High  RxVelocityTargetValue=0  RxVelocityTargetValueUnits=deg/s  RyEquilibriumPosition=0  RyEquilibriumPositionUnits=deg  RySpringStiffness=0  RySpringStiffnessUnits=N*m/deg  RyDampingCoefficient=0  RyDampingCoefficientUnits=N*m/(deg/s)  RyTorqueActuationMode=NoTorque  RyMotionActuationMode=ComputedMotion  RySensePosition=off  RySenseVelocity=off  RySenseAcceleration=off  RySenseTorqueForce=off  RySenseLowerLimitTorqueForce=off  RySenseUpperLimitTorqueForce=off  RyLowerLimitSpecify=off  RyLowerLimitBound=-90  RyLowerLimitBoundUnits=deg  RyLowerLimitStiffness=1e4  RyLowerLimitStiffnessUnits=N*m/deg  RyLowerLimitDamping=10  RyLowerLimitDampingUnits=N*m/(deg/s)  RyLowerLimitTransitionRegionWidth=0.1  RyLowerLimitTransitionRegionWidthUnits=deg  RyUpperLimitSpecify=off  RyUpperLimitBound=90  RyUpperLimitBoundUnits=deg  RyUpperLimitStiffness=1e4  RyUpperLimitStiffnessUnits=N*m/deg  RyUpperLimitDamping=10  RyUpperLimitDampingUnits=N*m/(deg/s)  RyUpperLimitTransitionRegionWidth=0.1  RyUpperLimitTransitionRegionWidthUnits=deg  RyPositionTargetSpecify=off  RyPositionTargetPriority=High  RyPositionTargetValue=0  RyPositionTargetValueUnits=deg  RyVelocityTargetSpecify=off  RyVelocityTargetPriority=High  RyVelocityTargetValue=0  RyVelocityTargetValueUnits=deg/s  RzEquilibriumPosition=0  RzEquilibriumPositionUnits=deg  RzSpringStiffness=0  RzSpringStiffnessUnits=N*m/deg  RzDampingCoefficient=0  RzDampingCoefficientUnits=N*m/(deg/s)  RzTorqueActuationMode=NoTorque  RzMotionActuationMode=ComputedMotion  RzSensePosition=off  RzSenseVelocity=off  RzSenseAcceleration=off  RzSenseTorqueForce=off  RzSenseLowerLimitTorqueForce=off  RzSenseUpperLimitTorqueForce=off  RzLowerLimitSpecify=off  RzLowerLimitBound=-90  RzLowerLimitBoundUnits=deg  RzLowerLimitStiffness=1e4  RzLowerLimitStiffnessUnits=N*m/deg  RzLowerLimitDamping=10  RzLowerLimitDampingUnits=N*m/(deg/s)  RzLowerLimitTransitionRegionWidth=0.1  RzLowerLimitTransitionRegionWidthUnits=deg  RzUpperLimitSpecify=off  RzUpperLimitBound=90  RzUpperLimitBoundUnits=deg  RzUpperLimitStiffness=1e4  RzUpperLimitStiffnessUnits=N*m/deg  RzUpperLimitDamping=10  RzUpperLimitDampingUnits=N*m/(deg/s)  RzUpperLimitTransitionRegionWidth=0.1  RzUpperLimitTransitionRegionWidthUnits=deg  RzPositionTargetSpecify=off  RzPositionTargetPriority=High  RzPositionTargetValue=0  RzPositionTargetValueUnits=deg  RzVelocityTargetSpecify=off  RzVelocityTargetPriority=High  RzVelocityTargetValue=0  RzVelocityTargetValueUnits=deg/s
  World Frame : sm_lib/Frames and Transforms/World Frame
  sacrum : sm_lib/Body Elements/File Solid  ExtGeomFileName=C:\Users\siril\OneDrive\Desktop\TIM-Control\Matlab\Simscape models\CAD - with COM\SymmetricModel\sacrum.step  UnitType=FromFile  ExtGeomFileUnits=m  StepReaderType=HEX  ExportConvexHullGeometry=off  InertiaType=CalculateFromGeometry  Mass=1  MassUnits=kg  CenterOfMass=[0 0 0]  CenterOfMassUnits=m  MomentsOfInertia=[1 1 1]  MomentsOfInertiaUnits=kg*m^2  ProductsOfInertia=[0 0 0]  ProductsOfInertiaUnits=kg*m^2  BasedOnType=Density  Density=0.182  DensityUnits=g/cm^3  DoExposeReferenceFrame=on  SerializedFrames=<Frames><Frame><Id>Frame1</Id><Value><Name>To L5</Name><Origin><Source>GeometricFeature</Source><FeatureName>planar surface 14566</FeatureName></Origin><PrimaryAxis><DefinedDirection>+Z</DefinedDirection><Source>GeometricFeature</Source><SourceDirection>+Z</SourceDirection><FeatureName>planar surface 14566</FeatureName></PrimaryAxis><SecondaryAxis><DefinedDirection>+X</DefinedDirection><Source>ReferenceFrame</Source><SourceDirection>+X</SourceDirection><FeatureName></FeatureName></SecondaryAxis></Value></Frame><Frame><Id>Frame2</Id><Value><Name>To Right Abdominal Muscle</Name><Origin><Source>GeometricFeature</Source><FeatureName>planar surface 54</FeatureName></Origin><PrimaryAxis><DefinedDirection>+Z</DefinedDirection><Source>ReferenceFrame</Source><SourceDirection>+Z</SourceDirection><FeatureName></FeatureName></PrimaryAxis><SecondaryAxis><DefinedDirection>+X</DefinedDirection><Source>ReferenceFrame</Source><SourceDirection>+X</SourceDirection><FeatureName></FeatureName></SecondaryAxis></Value></Frame><Frame><Id>Frame3</Id><Value><Name>To Left Abdominal Muscle</Name><Origin><Source>GeometricFeature</Source><FeatureName>planar surface 7390</FeatureName></Origin><PrimaryAxis><DefinedDirection>+Z</DefinedDirection><Source>ReferenceFrame</Source><SourceDirection>+Z</SourceDirection><FeatureName></FeatureName></PrimaryAxis><SecondaryAxis><DefinedDirection>+X</DefinedDirection><Source>ReferenceFrame</Source><SourceDirection>+X</SourceDirection><FeatureName></FeatureName></SecondaryAxis></Value></Frame><Frame><Id>Frame4</Id><Value><Name>To Right Back Muscle</Name><Origin><Source>GeometricFeature</Source><FeatureName>planar surface 26</FeatureName></Origin><PrimaryAxis><DefinedDirection>+Z</DefinedDirection><Source>ReferenceFrame</Source><SourceDirection>+Z</SourceDirection><FeatureName></FeatureName></PrimaryAxis><SecondaryAxis><DefinedDirection>+X</DefinedDirection><Source>ReferenceFrame</Source><SourceDirection>+X</SourceDirection><FeatureName></FeatureName></SecondaryAxis></Value></Frame><Frame><Id>Frame5</Id><Value><Name>To Left Back Muscle</Name><Origin><Source>GeometricFeature</Source><FeatureName>planar surface 7362</FeatureName></Origin><PrimaryAxis><DefinedDirection>+Z</DefinedDirection><Source>ReferenceFrame</Source><SourceDirection>+Z</SourceDirection><FeatureName></FeatureName></PrimaryAxis><SecondaryAxis><DefinedDirection>+X</DefinedDirection><Source>ReferenceFrame</Source><SourceDirection>+X</SourceDirection><FeatureName></FeatureName></SecondaryAxis></Value></Frame><Frame><Id>Frame6</Id><Value><Name>To Right Transverse1 Muscle</Name><Origin><Source>GeometricFeature</Source><FeatureName>planar surface 19</FeatureName></Origin><PrimaryAxis><DefinedDirection>+Z</DefinedDirection><Source>ReferenceFrame</Source><SourceDirection>+Z</SourceDirection><FeatureName></FeatureName></PrimaryAxis><SecondaryAxis><DefinedDirection>+X</DefinedDirection><Source>ReferenceFrame</Source><SourceDirection>+X</SourceDirection><FeatureName></FeatureName></SecondaryAxis></Value></Frame><Frame><Id>Frame7</Id><Value><Name>To Right Transverse2 Muscle</Name><Origin><Source>GeometricFeature</Source><FeatureName>planar surface 5</FeatureName></Origin><PrimaryAxis><DefinedDirection>+Z</DefinedDirection><Source>ReferenceFrame</Source><SourceDirection>+Z</SourceDirection><FeatureName></FeatureName></PrimaryAxis><SecondaryAxis><DefinedDirection>+X</DefinedDirection><Source>ReferenceFrame</Source><SourceDirection>+X</SourceDirection><FeatureName></FeatureName></SecondaryAxis></Value></Frame><Frame><Id>Frame8</Id><Value><Name>To Left Transverse1 Muscle</Name><Origin><Source>GeometricFeature</Source><FeatureName>planar surface 7355</FeatureName></Origin><PrimaryAxis><DefinedDirection>+Z</DefinedDirection><Source>ReferenceFrame</Source><SourceDirection>+Z</SourceDirection><FeatureName></FeatureName></PrimaryAxis><SecondaryAxis><DefinedDirection>+X</DefinedDirection><Source>ReferenceFrame</Source><SourceDirection>+X</SourceDirection><FeatureName></FeatureName></SecondaryAxis></Value></Frame><Frame><Id>Frame9</Id><Value><Name>To Left Transverse2 Muscle</Name><Origin><Source>GeometricFeature</Source><FeatureName>planar surface 7341</FeatureName></Origin><PrimaryAxis><DefinedDirection>+Z</DefinedDirection><Source>ReferenceFrame</Source><SourceDirection>+Z</SourceDirection><FeatureName></FeatureName></PrimaryAxis><SecondaryAxis><DefinedDirection>+X</DefinedDirection><Source>ReferenceFrame</Source><SourceDirection>+X</SourceDirection><FeatureName></FeatureName></SecondaryAxis></Value></Frame><Frame><Id>Frame10</Id><Value><Name>For Plumbline Evaluation</Name><Origin><Source>GeometricFeature</Source><FeatureName>planar surface 14546</FeatureName></Origin><PrimaryAxis><DefinedDirection>+Z</DefinedDirection><Source>ReferenceFrame</Source><SourceDirection>+Z</SourceDirection><FeatureName></FeatureName></PrimaryAxis><SecondaryAxis><DefinedDirection>+X</DefinedDirection><Source>ReferenceFrame</Source><SourceDirection>+X</SourceDirection><FeatureName></FeatureName></SecondaryAxis></Value></Frame><Frame><Id>Frame11</Id><Value><Name>To Abdomen - Right</Name><Origin><Source>GeometricFeature</Source><FeatureName>planar surface 2380</FeatureName></Origin><PrimaryAxis><DefinedDirection>+Z</DefinedDirection><Source>ReferenceFrame</Source><SourceDirection>+Z</SourceDirection><FeatureName></FeatureName></PrimaryAxis><SecondaryAxis><DefinedDirection>+X</DefinedDirection><Source>ReferenceFrame</Source><SourceDirection>+X</SourceDirection><FeatureName></FeatureName></SecondaryAxis></Value></Frame><Frame><Id>Frame12</Id><Value><Name>To Abdomen - Left</Name><Origin><Source>GeometricFeature</Source><FeatureName>planar surface 9716</FeatureName></Origin><PrimaryAxis><DefinedDirection>+Z</DefinedDirection><Source>ReferenceFrame</Source><SourceDirection>+Z</SourceDirection><FeatureName></FeatureName></PrimaryAxis><SecondaryAxis><DefinedDirection>+X</DefinedDirection><Source>ReferenceFrame</Source><SourceDirection>+X</SourceDirection><FeatureName></FeatureName></SecondaryAxis></Value></Frame><Frame><Id>Frame13</Id><Value><Name>To L5 ISL</Name><Origin><Source>GeometricFeature</Source><FeatureName>point 22330</FeatureName></Origin><PrimaryAxis><DefinedDirection>+Z</DefinedDirection><Source>ReferenceFrame</Source><SourceDirection>+Z</SourceDirection><FeatureName></FeatureName></PrimaryAxis><SecondaryAxis><DefinedDirection>+X</DefinedDirection><Source>ReferenceFrame</Source><SourceDirection>+X</SourceDirection><FeatureName></FeatureName></SecondaryAxis></Value></Frame><Frame><Id>Frame14</Id><Value><Name>To L5 SSL</Name><Origin><Source>GeometricFeature</Source><FeatureName>point 44660</FeatureName></Origin><PrimaryAxis><DefinedDirection>+Z</DefinedDirection><Source>ReferenceFrame</Source><SourceDirection>+Z</SourceDirection><FeatureName></FeatureName></PrimaryAxis><SecondaryAxis><DefinedDirection>+X</DefinedDirection><Source>ReferenceFrame</Source><SourceDirection>+X</SourceDirection><FeatureName></FeatureName></SecondaryAxis></Value></Frame><Frame><Id>Frame15</Id><Value><Name>To Right L5 ITL</Name><Origin><Source>GeometricFeature</Source><FeatureName>point 13718</FeatureName></Origin><PrimaryAxis><DefinedDirection>+Z</DefinedDirection><Source>ReferenceFrame</Source><SourceDirection>+Z</SourceDirection><FeatureName></FeatureName></PrimaryAxis><SecondaryAxis><DefinedDirection>+X</DefinedDirection><Source>ReferenceFrame</Source><SourceDirection>+X</SourceDirection><FeatureName></FeatureName></SecondaryAxis></Value></Frame><Frame><Id>Frame16</Id><Value><Name>To left L5 ITL</Name><Origin><Source>GeometricFeature</Source><FeatureName>point 36305</FeatureName></Origin><PrimaryAxis><DefinedDirection>+Z</DefinedDirection><Source>ReferenceFrame</Source><SourceDirection>+Z</SourceDirection><FeatureName></FeatureName></PrimaryAxis><SecondaryAxis><DefinedDirection>+X</DefinedDirection><Source>ReferenceFrame</Source><SourceDirection>+X</SourceDirection><FeatureName></FeatureName></SecondaryAxis></Value></Frame><Frame><Id>Frame17</Id><Value><Name>Sacrum COM</Name><Origin><Source>CenterOfMassFrame</Source><FeatureName></FeatureName></Origin><PrimaryAxis><DefinedDirection>+Z</DefinedDirection><Source>ReferenceFrame</Source><SourceDirection>+Z</SourceDirection><FeatureName></FeatureName></PrimaryAxis><SecondaryAxis><DefinedDirection>+X</DefinedDirection><Source>ReferenceFrame</Source><SourceDirection>+X</SourceDirection><FeatureName></FeatureName></SecondaryAxis></Value></Frame></Frames>  GraphicType=FromGeometry  MarkerShape=Sphere  MarkerSize=10  GraphicVisPropType=SimpleVisualProperties  GraphicDiffuseColor=[0.5 0.5 0.5]  GraphicSpecularColor=[0.5 0.5 0.5 1.0]  GraphicAmbientColor=[0.15 0.15 0.15 1.0]  GraphicEmissiveColor=[0.0 0.0 0.0 1.0]  GraphicShininess=75  GraphicOpacity=1.0
  wires:
  PS-Simulink Converter2/1 -> Gain/1  "x"
  PS-Simulink Converter3/1 -> Gain1/1  "y"
  PS-Simulink Converter4/1 -> Gain2/1  "z"
  Gain/1 -> Check X Bounds/1, Scope9/1, Plumbline X distance (cm)/1  "x"
  Gain1/1 -> Scope9/2, Check Y Bounds/1, Plumbline Y distance (cm)/1  "y"
  Gain2/1 -> Plumbline Z distance (cm)/1, Scope9/3
  Ramp/1 -> Simulink-PS Converter1/1
  PS-Simulink Converter9/1 -> Radians to Degrees4/1
  Radians to Degrees4/1 -> Add/1
  Add/1 -> Gain6/1
  Gain6/1 -> Check Flexion Angle/1, Scope1/1, L1-S1 FE Simscape/1  "L1-S1 FE Simscape Rotation"
  Gain7/1 -> L1-S1 FE Simscape/2  "L1-S1 FE Simscape Moment"
  Constant3/1 -> Add1/2
  Gain4/1 -> L1-S1 LB Simscape/2  "L1-S1 LB Simscape Moment"
  Radians to Degrees1/1 -> Add1/1
  Gain3/1 -> Scope/1, L1-S1 LB Simscape/1  "L1-S1 LB Simscape Rotation"
  Add1/1 -> Gain3/1
  PS-Simulink Converter1/1 -> Radians to Degrees1/1
  Constant4/1 -> Add2/2
  Gain8/1 -> L1-S1 AR Simscape/2  "L1-S1 AR Simscape Moment"
  Radians to Degrees2/1 -> Add2/1
  Gain5/1 -> Scope3/1, L1-S1 AR Simscape/1  "L1-S1 AR Simscape Rotation"
  Add2/1 -> Gain5/1
  PS-Simulink Converter5/1 -> Radians to Degrees2/1
  Moment_LB/1 -> Gain4/1, Simulink-PS Converter3/1
  Moment_AR/1 -> Gain8/1, Simulink-PS Converter4/1
  Moment_FE/1 -> Scope2/1, Simulink-PS Converter2/1, Gain7/1
  Constant2/1 -> Add/2
  PS-Simulink Converter8/1 -> Add3/2
  PS-Simulink Converter10/1 -> Add3/1
  Add3/1 -> Gain9/1, IAP Extensor Torque at L3/1
  Gain9/1 -> Display/1
  connections:
  L5/RConn1 -- L4/LConn1
  L3/LConn1 -- L4/RConn1
  L3/RConn1 -- L2/LConn1
  L2/RConn1 -- L1/LConn1
  sacrum/RConn1 -- IAP - Internal Springs Model/RConn6 -- World Frame/RConn1 -- Mechanism Configuration/RConn1 -- Solver Configuration/RConn1
  PS-Simulink Converter2/LConn1 -- T1-S1 Bushing Joint/RConn2
  PS-Simulink Converter3/LConn1 -- T1-S1 Bushing Joint/RConn3
  PS-Simulink Converter4/LConn1 -- T1-S1 Bushing Joint/RConn4
  L1-S1 Bushing Joint/RConn1 -- L1/RConn1 -- IAP - Individual Forces Model/LConn1 -- IAP - Internal Springs Model/LConn1 -- Right T Spine/LConn1 -- Left T Spine/LConn1
  T1-S1 Bushing Joint/RConn1 -- Right T Spine/RConn3 -- Flexion force at T1/RConn1
  sacrum/RConn2 -- Muscle Forces/LConn1
  sacrum/LConn2 -- Muscle Forces/LConn2
  sacrum/RConn3 -- Muscle Forces/LConn3
  Muscle Forces/LConn4 -- sacrum/LConn3
  sacrum/RConn4 -- Muscle Forces/LConn5
  sacrum/LConn4 -- Muscle Forces/LConn6
  Muscle Forces/LConn7 -- sacrum/RConn5
  sacrum/LConn5 -- Muscle Forces/LConn8
  Left T Spine/LConn2 -- Muscle Forces/RConn6
  Left T Spine/RConn2 -- Muscle Forces/RConn7
  Left T Spine/LConn3 -- Muscle Forces/RConn8
  sacrum/LConn6 -- L1-S1 Bushing Joint/LConn1 -- T1-S1 Bushing Joint/LConn1
  Simulink-PS Converter1/RConn1 -- Flexion force at T1/LConn1
  Simulink-PS Converter2/RConn1 -- Pure FE Moment at L1 COM/LConn1
  Pure FE Moment at L1 COM/RConn1 -- Pure AR Moment at L1 COM/RConn1 -- Pure LB Moment at L1 COM/RConn1 -- L1/RConn8
  L1/RConn2 -- L1-L2 FE/LConn2
  L1/RConn3 -- PS-Simulink Converter10/LConn1 -- L1-L2 FE/LConn1
  L1-S1 Bushing Joint/RConn2 -- PS-Simulink Converter9/LConn1
  L5/RConn2 -- L5-S1 FE/LConn1
  L5/RConn3 -- L5-S1 FE/LConn2
  L4/RConn2 -- L4-L5  FE/LConn1
  L4/RConn3 -- L4-L5  FE/LConn2
  L3-L4 FE/LConn2 -- L3/RConn3
  L3-L4 FE/LConn1 -- L3/RConn2
  L2-L3 FE/LConn2 -- L2/RConn2
  L2-L3 FE/LConn1 -- PS-Simulink Converter8/LConn1 -- L2/RConn3
  L4-L5  LB/LConn2 -- L4/RConn4
  L1-L2 LB/LConn2 -- L1/RConn4
  L3-L4 LB/LConn2 -- L3/RConn4
  L2-L3 LB/LConn2 -- L2/RConn4
  L3-L4 LB/LConn1 -- L3/RConn5
  L4-L5  LB/LConn1 -- L4/RConn5
  L2-L3 LB/LConn1 -- L2/RConn5
  L1-L2 LB/LConn1 -- L1/RConn5
  L5-S1 LB/LConn1 -- L5/RConn5
  L5/RConn4 -- L5-S1 LB/LConn2
  L3-L4 AR/LConn1 -- L3/RConn7
  L2-L3 AR/LConn1 -- L2/RConn7
  L3-L4 AR/LConn2 -- L3/RConn6
  L1-L2 AR/LConn1 -- L1/RConn7
  L2-L3 AR/LConn2 -- L2/RConn6
  L1-L2 AR/LConn2 -- L1/RConn6
  L5-S1 AR/LConn2 -- L5/RConn6
  L5-S1 AR/LConn1 -- L5/RConn7
  PS-Simulink Converter1/LConn1 -- L1-S1 Bushing Joint/RConn3
  PS-Simulink Converter5/LConn1 -- L1-S1 Bushing Joint/RConn4
  Pure LB Moment at L1 COM/LConn1 -- Simulink-PS Converter3/RConn1
  Simulink-PS Converter4/RConn1 -- Pure AR Moment at L1 COM/LConn1
  L4/RConn6 -- L4-L5  AR/LConn2
  L4/RConn7 -- L4-L5  AR/LConn1
  IAP - Individual Forces Model/RConn1 -- IAP - Internal Springs Model/RConn1 -- L5/RConn9
  IAP - Individual Forces Model/RConn2 -- IAP - Internal Springs Model/RConn2 -- L4/RConn9
  IAP - Individual Forces Model/RConn3 -- IAP - Internal Springs Model/RConn3 -- L2/RConn9
  IAP - Individual Forces Model/RConn4 -- IAP - Internal Springs Model/RConn4 -- L3/RConn9
  IAP - Individual Forces Model/RConn5 -- IAP - Internal Springs Model/RConn5 -- L1/RConn9
  Muscle Forces/RConn5 -- Left T Spine/RConn1
  Muscle Forces/RConn4 -- Right T Spine/RConn2
  Muscle Forces/RConn3 -- Right T Spine/LConn3
  Muscle Forces/RConn2 -- Right T Spine/LConn2
  Muscle Forces/RConn1 -- Right T Spine/RConn1
  L5/RConn10 -- Interspinous Ligaments/LConn2
  Interspinous Ligaments/LConn3 -- L4/RConn10
  Interspinous Ligaments/LConn4 -- L2/RConn10
  Interspinous Ligaments/LConn5 -- L5/RConn11
  Interspinous Ligaments/LConn6 -- L4/RConn11
  Interspinous Ligaments/LConn7 -- L3/RConn10
  Interspinous Ligaments/LConn8 -- L2/RConn11
  Interspinous Ligaments/LConn9 -- L3/RConn11
  Interspinous Ligaments/LConn10 -- L1/RConn10
  Interspinous Ligaments/LConn1 -- sacrum/RConn7
  Supraspinous Ligaments/LConn1 -- L5/RConn12
  Supraspinous Ligaments/LConn2 -- L4/RConn12 -- Sagittaal Kinematics Readings/RConn4
  Supraspinous Ligaments/LConn3 -- Sagittaal Kinematics Readings/RConn1 -- L2/RConn12
  L5/RConn13 -- Sagittaal Kinematics Readings/RConn5 -- Supraspinous Ligaments/LConn4
  Supraspinous Ligaments/LConn5 -- L4/RConn13
  Supraspinous Ligaments/LConn6 -- L3/RConn12
  Supraspinous Ligaments/LConn7 -- L2/RConn13
  Supraspinous Ligaments/LConn8 -- Sagittaal Kinematics Readings/RConn2 -- L3/RConn13
  Supraspinous Ligaments/LConn9 -- Sagittaal Kinematics Readings/RConn3 -- L1/RConn11
  sacrum/LConn8 -- Sagittaal Kinematics Readings/LConn1 -- Supraspinous Ligaments/LConn10
  Left and Right Intertransverse Ligaments/LConn2 -- L5/RConn14
  Left and Right Intertransverse Ligaments/LConn3 -- L4/RConn14
  L3/RConn14 -- Left and Right Intertransverse Ligaments/LConn4
  L2/RConn14 -- Left and Right Intertransverse Ligaments/LConn5
  Left and Right Intertransverse Ligaments/LConn6 -- L5/RConn15
  Left and Right Intertransverse Ligaments/LConn7 -- L4/RConn15
  L3/RConn15 -- Left and Right Intertransverse Ligaments/LConn8
  L2/RConn15 -- Left and Right Intertransverse Ligaments/LConn9
  Left and Right Intertransverse Ligaments/LConn10 -- L5/RConn16
  L4/RConn16 -- Left and Right Intertransverse Ligaments/LConn11
  L3/RConn16 -- Left and Right Intertransverse Ligaments/LConn12
  L2/RConn16 -- Left and Right Intertransverse Ligaments/LConn13
  L1/RConn12 -- Left and Right Intertransverse Ligaments/LConn14
  Left and Right Intertransverse Ligaments/LConn15 -- L5/RConn17
  L4/RConn17 -- Left and Right Intertransverse Ligaments/LConn16
  L3/RConn17 -- Left and Right Intertransverse Ligaments/LConn17
  L2/RConn17 -- Left and Right Intertransverse Ligaments/LConn18
  L1/RConn13 -- Left and Right Intertransverse Ligaments/LConn19
  Left and Right Intertransverse Ligaments/LConn20 -- sacrum/LConn9
  Left and Right Intertransverse Ligaments/LConn1 -- sacrum/RConn8
  IAP - Internal Springs Model/RConn7 -- sacrum/RConn9
  sacrum/LConn1 -- L5/LConn1
  Sagittaal Kinematics Readings/RConn6 -- Right T Spine/LConn4
  Sagittaal Kinematics Readings/RConn7 -- Right T Spine/RConn4
  Sagittaal Kinematics Readings/RConn8 -- Right T Spine/LConn5
  Sagittaal Kinematics Readings/RConn9 -- Right T Spine/RConn5
